simulink model "sit2 (1)"  (R2018b)
settings: Solver=VariableStepAuto  StartTime=0.0  StopTime=10.0  RelTol=1e-3
values from neighbouring files (symbols this model uses):
  B = 25    [WORKSPACE (1).m]
  F = 8    [WORKSPACE (1).m]
  K = 16    [WORKSPACE (1).m]
  M = 2    [WORKSPACE (1).m]
settings Model: Creator=student  LastModifiedBy=student

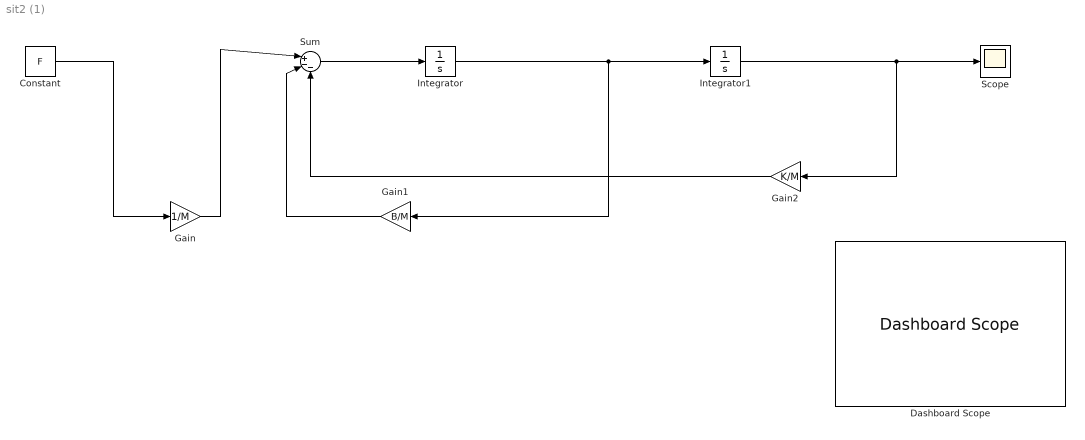
== system sit2 (1) ==
  Constant : Constant  Value=F
  Dashboard Scope : DashboardScope  WebBlockId=10
  Gain : Gain  Gain=1/M
  Gain1 : Gain  Gain=B/M
  Gain2 : Gain  Gain=K/M
  Integrator : Integrator
  Integrator1 : Integrator
  Scope : Scope
  Sum : Sum  Inputs=|+--
  wires:
  Constant/1 -> Gain/1
  Gain/1 -> Sum/1
  Gain1/1 -> Sum/2
  Gain2/1 -> Sum/3
  Sum/1 -> Integrator/1
  Integrator/1 -> Gain1/1, Integrator1/1
  Integrator1/1 -> Gain2/1, Scope/1
